simulink model "sysp3"  (R2023a)
settings: Solver=ode15s  StartTime=0.0  StopTime=10  MaxStep=1E-3  RelTol=1e-3
settings Model: Creator=Ariel  LastModifiedBy=Ariel
settings SolverCC: MaxConsecutiveZCs=10
settings DataIOCC: ReturnWorkspaceOutputs=off  TimeSaveName=t
settings DebuggingCC: AlgebraicLoopMsg=none  ArtificialAlgebraicLoopMsg=none  MaxConsecutiveZCsMsg=none  ModelReferenceExtraNoncontSigs=none  OperatingPointInterfaceChecksumMismatchMsg=none

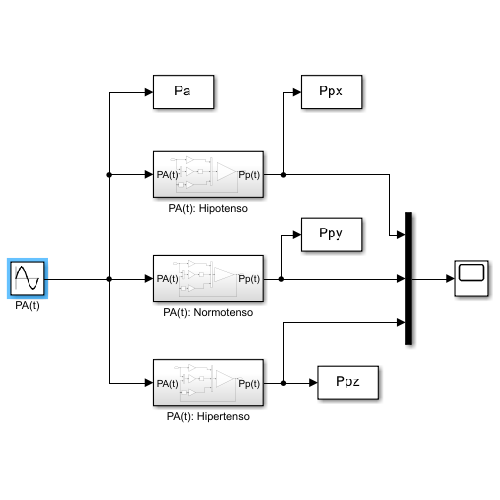
[thumbnail: Simulink's stored preview of the top-level diagram]
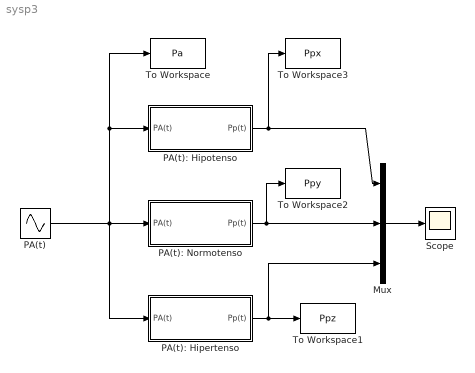
== system sysp3 ==
  Mux : Mux  Inputs=3
  PA(t) : Sin  Bias=0.8  Frequency=2*pi*95/60  SampleTime=0
  PA(t): Hipertenso : Subsystem
  PA(t): Hipotenso : Subsystem
  PA(t): Normotenso : Subsystem
  Scope : Scope
  To Workspace : ToWorkspace  VariableName=Pa  SaveFormat=Timeseries  SampleTime=-1
  To Workspace1 : ToWorkspace  VariableName=Ppz  SaveFormat=Timeseries  SampleTime=-1
  To Workspace2 : ToWorkspace  VariableName=Ppy  SaveFormat=Timeseries  SampleTime=-1
  To Workspace3 : ToWorkspace  VariableName=Ppx  SaveFormat=Timeseries  SampleTime=-1
  wires:
  Mux/1 -> Scope/1
  PA(t)/1 -> PA(t): Hipertenso/1(PA(t)), To Workspace/1, PA(t): Hipotenso/1(PA(t)), PA(t): Normotenso/1(PA(t))
  PA(t): Hipotenso/1(Pp(t)) -> Mux/1, To Workspace3/1
  PA(t): Hipertenso/1(Pp(t)) -> To Workspace1/1, Mux/3
  PA(t): Normotenso/1(Pp(t)) -> Mux/2, To Workspace2/1

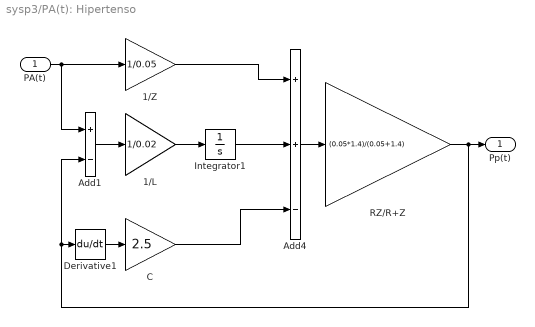
== system sysp3/PA(t): Hipertenso ==
  PA(t) : Inport
  1/L : Gain  Gain=1/0.02
  1/Z : Gain  Gain=1/0.05
  Add1 : Sum  Inputs=+-
  Add4 : Sum  Inputs=++-
  C : Gain  Gain=2.5
  Derivative1 : Derivative
  Integrator1 : Integrator
  RZ/R+Z : Gain  Gain=(0.05*1.4)/(0.05+1.4)
  Pp(t) : Outport
  wires:
  PA(t)/1 -> 1/Z/1, Add1/1
  1/Z/1 -> Add4/1
  1/L/1 -> Integrator1/1
  Add1/1 -> 1/L/1
  Integrator1/1 -> Add4/2
  Add4/1 -> RZ/R+Z/1
  RZ/R+Z/1 -> Derivative1/1, Add1/2, Pp(t)/1
  Derivative1/1 -> C/1
  C/1 -> Add4/3

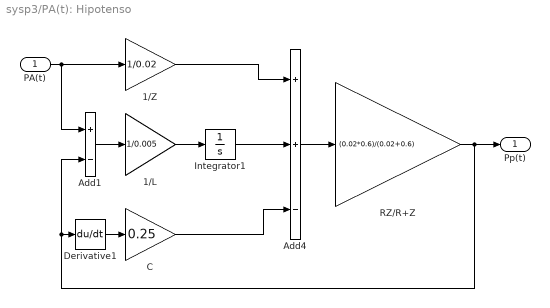
== system sysp3/PA(t): Hipotenso ==
  PA(t) : Inport
  1/L : Gain  Gain=1/0.005
  1/Z : Gain  Gain=1/0.02
  Add1 : Sum  Inputs=+-
  Add4 : Sum  Inputs=++-
  C : Gain  Gain=0.25
  Derivative1 : Derivative
  Integrator1 : Integrator
  RZ/R+Z : Gain  Gain=(0.02*0.6)/(0.02+0.6)
  Pp(t) : Outport
  wires:
  PA(t)/1 -> 1/Z/1, Add1/1
  1/Z/1 -> Add4/1
  1/L/1 -> Integrator1/1
  Add1/1 -> 1/L/1
  Integrator1/1 -> Add4/2
  C/1 -> Add4/3
  Add4/1 -> RZ/R+Z/1
  RZ/R+Z/1 -> Pp(t)/1, Derivative1/1, Add1/2
  Derivative1/1 -> C/1

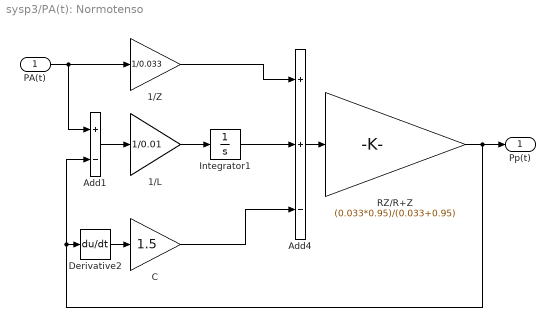
== system sysp3/PA(t): Normotenso ==
  PA(t) : Inport
  1/L : Gain  Gain=1/0.01
  1/Z : Gain  Gain=1/0.033
  Add1 : Sum  Inputs=+-
  Add4 : Sum  Inputs=++-
  C : Gain  Gain=1.5
  Derivative2 : Derivative
  Integrator1 : Integrator
  RZ/R+Z : Gain  Gain=(0.033*0.95)/(0.033+0.95)
  Pp(t) : Outport
  wires:
  PA(t)/1 -> 1/Z/1, Add1/1
  1/Z/1 -> Add4/1
  1/L/1 -> Integrator1/1
  Add1/1 -> 1/L/1
  Integrator1/1 -> Add4/2
  Add4/1 -> RZ/R+Z/1
  RZ/R+Z/1 -> Derivative2/1, Add1/2, Pp(t)/1
  Derivative2/1 -> C/1
  C/1 -> Add4/3
